simulink model "Simulacion (1)"  (R2024a)
settings: Solver=VariableStepAuto  StartTime=0.0  StopTime=30  RelTol=1e-3
values from neighbouring files (symbols this model uses):
  F = 5    [V1_Control.m]
  g = 9.81    [V1_Control.m]
  J = 0.01    [V1_Control.m]
  L = 0.3    [V1_Control.m]
  M = 0.301    [V1_Control.m]
  m = 0.101    [V1_Control.m]
  S = 0.00001    (= 1e-05)    [V1_Control.m]
  Tm = 0.01    [V1_Control.m]
libraries: simulink x1
settings Model: Creator=Miran  LastModifiedBy=Miran

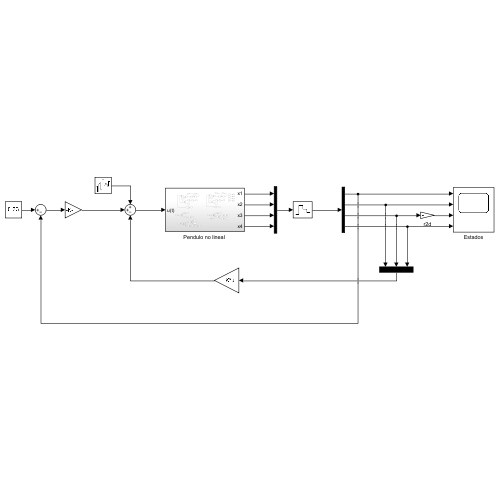
[thumbnail: Simulink's stored preview of the top-level diagram]
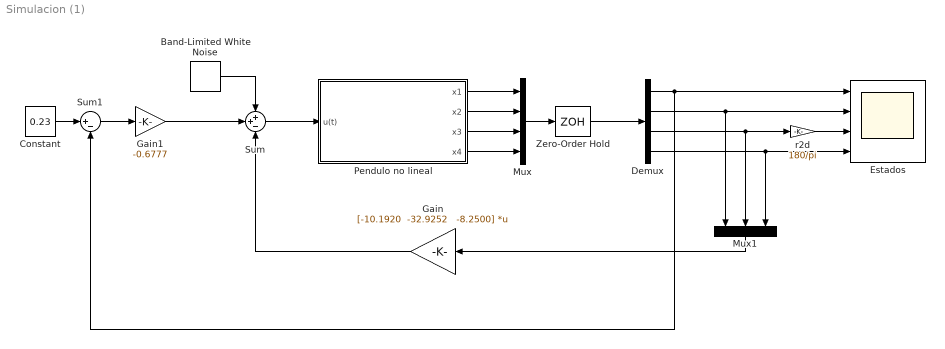
== system Simulacion (1) ==
  Band-Limited White Noise : simulink/Sources/Band-Limited White Noise  Cov=[0.001]  Ts=Tm  seed=[23341]
  Constant : Constant  Value=0.23
  Demux : Demux
  Estados : Scope  NumInputPorts=4
  Gain : Gain  Gain="[-10.1920  -32.9252   -8.2500]"  Multiplication=Matrix(K*u)
  Gain1 : Gain  Gain=-0.6777
  Mux : Mux
  Mux1 : Mux  Inputs=3
  "Pendulo no lineal " : Subsystem
  Sum : Sum  Inputs=++-
  Sum1 : Sum  Inputs=|+-
  Zero-Order Hold : ZeroOrderHold  SampleTime=Tm
  r2d : Gain  Gain=180/pi
  wires:
  r2d/1 -> Estados/3
  Constant/1 -> Sum1/1
  Mux1/1 -> Gain/1
  Sum1/1 -> Gain1/1
  Demux/3 -> Mux1/2, r2d/1
  Demux/2 -> Mux1/1, Estados/2
  Demux/1 -> Estados/1, Sum1/2
  Demux/4 -> Mux1/3, Estados/4
  Mux/1 -> Zero-Order Hold/1
  Zero-Order Hold/1 -> Demux/1
  "Pendulo no lineal "/1(x1) -> Mux/1
  "Pendulo no lineal "/2(x2) -> Mux/2
  "Pendulo no lineal "/3(x3) -> Mux/3
  "Pendulo no lineal "/4(x4) -> Mux/4
  Sum/1 -> "Pendulo no lineal "/1(u(t))
  Gain/1 -> Sum/3
  Gain1/1 -> Sum/2
  Band-Limited White Noise/1 -> Sum/1

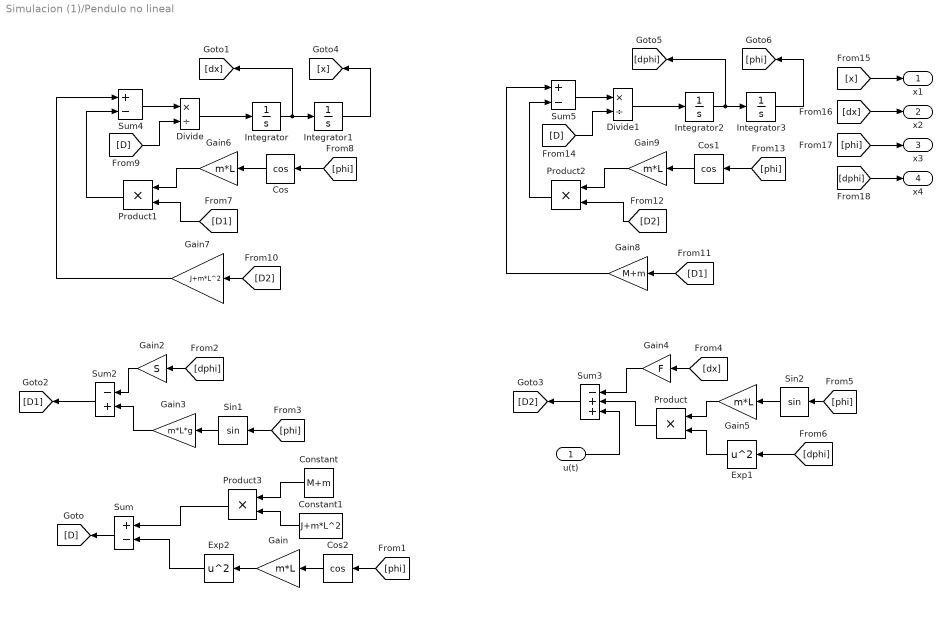
== system Simulacion (1)/Pendulo no lineal  ==
  u(t) : Inport
  Constant : Constant  Value=M+m
  Constant1 : Constant  Value=J+m*L^2
  Cos : Trigonometry  Operator=cos
  Cos1 : Trigonometry  Operator=cos
  Cos2 : Trigonometry  Operator=cos
  Divide : Product  Inputs=*/  RndMeth=Zero  SaturateOnIntegerOverflow=on
  Divide1 : Product  Inputs=*/  RndMeth=Zero  SaturateOnIntegerOverflow=on
  Exp1 : Math  Operator=square
  Exp2 : Math  Operator=square
  Gain{,5..6,9} (4 alike) : Gain  Gain=m*L
  Gain2 : Gain  Gain=S
  Gain3 : Gain  Gain=m*L*g
  Gain4 : Gain  Gain=F
  Gain7 : Gain  Gain=J+m*L^2
  Gain8 : Gain  Gain=M+m
  Integrator : Integrator
  Integrator1 : Integrator  InitialCondition=0.23
  Integrator2 : Integrator  InitialCondition=0.1
  Integrator3 : Integrator  InitialCondition=0.06
  Product{,1..3} (4 alike) : Product
  Sin1 : Trigonometry
  Sin2 : Trigonometry
  Sum : Sum  Inputs=+-
  Sum2 : Sum  Inputs=-+
  Sum3 : Sum  Inputs=-++
  Sum4 : Sum  Inputs=+-
  Sum5 : Sum  Inputs=+-
  x1 : Outport
  x2 : Outport  Port=2
  x3 : Outport  Port=3
  x4 : Outport  Port=4
  wires:
  Integrator/1 -> [dx], Integrator1/1
  Sum/1 -> [D]
  Divide/1 -> Integrator/1
  [dx] -> Gain4/1
  Gain4/1 -> Sum3/1
  [phi] -> x3/1
  [phi] -> Cos1/1
  [D] -> Divide1/2
  [D] -> Divide/2
  [phi] -> Sin2/1
  [dphi] -> x4/1
  Sin1/1 -> Gain3/1
  [dphi] -> Exp1/1
  Cos1/1 -> Gain9/1
  Gain2/1 -> Sum2/1
  [D2] -> Product2/2
  Gain9/1 -> Product2/1
  Integrator2/1 -> [dphi], Integrator3/1
  [dx] -> x2/1
  [phi] -> Sin1/1
  Sum2/1 -> [D1]
  Integrator1/1 -> [x]
  [D2] -> Gain7/1
  Product1/1 -> Sum4/2
  Sum5/1 -> Divide1/1
  [D1] -> Product1/2
  Integrator3/1 -> [phi]
  Sin2/1 -> Gain5/1
  u(t)/1 -> Sum3/3
  Product/1 -> Sum3/2
  Exp1/1 -> Product/2
  Product2/1 -> Sum5/2
  Sum3/1 -> [D2]
  [dphi] -> Gain2/1
  Divide1/1 -> Integrator2/1
  [D1] -> Gain8/1
  Gain5/1 -> Product/1
  Gain6/1 -> Product1/1
  Gain8/1 -> Sum5/1
  [x] -> x1/1
  Sum4/1 -> Divide/1
  Cos/1 -> Gain6/1
  [phi] -> Cos/1
  Gain7/1 -> Sum4/1
  Gain3/1 -> Sum2/2
  Constant/1 -> Product3/1
  Constant1/1 -> Product3/2
  Cos2/1 -> Gain/1
  [phi] -> Cos2/1
  Product3/1 -> Sum/1
  Gain/1 -> Exp2/1
  Exp2/1 -> Sum/2
